simulink model "Bomb"  (R2014a)
settings: Solver=ode45  StartTime=0.0  StopTime=30  RelTol=1e-3
settings Model: Creator=pc32  LastModifiedBy=marwan
settings DebuggingCC: UnderspecifiedInitializationDetection=Classic  StateNameClashWarn=warning

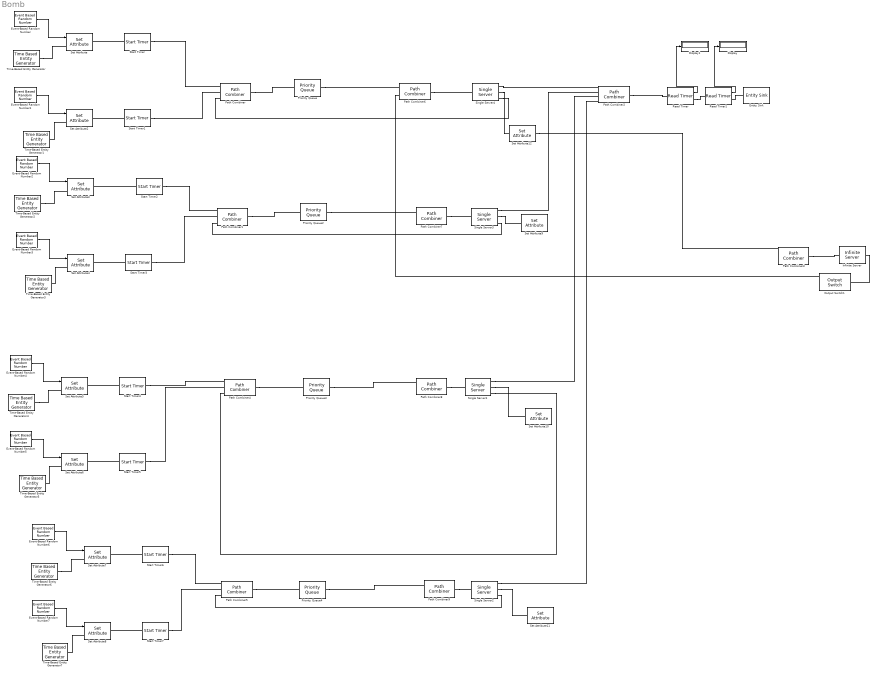
== system Bomb ==
  Display : Display
  Display1 : Display
  Entity Sink : EntitySink
  Event-Based Random Number : EventBasedRandomNumber  meanExp=1/100  Seed=40859
  Event-Based Random Number1 : EventBasedRandomNumber  meanExp=1/100  Seed=94546
  Event-Based Random Number2 : EventBasedRandomNumber  meanExp=1/100  Seed=3
  Event-Based Random Number3 : EventBasedRandomNumber  meanExp=1/100  Seed=4
  Event-Based Random Number4 : EventBasedRandomNumber  meanExp=1/100  Seed=44076
  Event-Based Random Number5 : EventBasedRandomNumber  meanExp=1/100  Seed=5
  Event-Based Random Number6 : EventBasedRandomNumber  meanExp=1/100  Seed=6
  Event-Based Random Number7 : EventBasedRandomNumber  meanExp=1/100  Seed=7
  Infinite Server : InfiniteServer  ServiceTime=0
  Output Switch1 : OutputSwitch  NumberOutputPorts=5  AttributeName=type
  Path Combiner{,1,4..5} (4 alike) : PathCombiner
  Path Combiner2 : PathCombiner  NumberInputPorts=4
  Path Combiner3 : PathCombiner  NumberInputPorts=4
  Path Combiner{6..9} (4 alike) : PathCombiner  NumberInputPorts=2
  Priority Queue{,2..4} (4 alike) : PriorityQueue  Capacity=inf  SortingAttributeName=priority
  Read Timer : ReadTimer  TimerTag=TP  TimerModeOption=Ignore  StatAverageTimeElapsed=on
      settings: OutputPortMap=o3
  Read Timer1 : ReadTimer  TimerTag=TS  TimerModeOption=Ignore  StatAverageTimeElapsed=on
      settings: OutputPortMap=o3
  Set Attribute{,3,5,7} (4 alike) : SetAttribute  AttributeName=ServTime|priority  AttributeFrom=Signal port|Dialog  AttributeValue=1|1  AttributeTreatAsVector=1|1  EvaluatedAttributeValue={ [];1}
  Set Attribute10 : SetAttribute  AttributeName=ch  AttributeValue=3  EvaluatedAttributeValue={ 3}
  Set Attribute11 : SetAttribute  AttributeName=ch  AttributeValue=4  EvaluatedAttributeValue={ 4}
  Set Attribute12 : SetAttribute  AttributeName=ch|priority  AttributeFrom=Dialog|Dialog  AttributeValue=1|2  AttributeTreatAsVector=1|1  EvaluatedAttributeValue={ 1;2}
  Set Attribute{2,4,6,8} (4 alike) : SetAttribute  AttributeName=ServTime|priority  AttributeFrom=Signal port|Dialog  AttributeValue=1|3  AttributeTreatAsVector=1|1  EvaluatedAttributeValue={ [];3}
  Set Attribute9 : SetAttribute  AttributeName=ch  AttributeValue=2  EvaluatedAttributeValue={ 2}
  Single Server{1..4} (4 alike) : SingleServer  ServiceTimeFrom=Attribute  ServiceTime=0  AttributeName=ServTime  PermitPreemption=on  SortingAttributeName=priority  WriteToAttribute=on  ResidualAttributeName=ServTime  EnableTOPort=on
  Start Timer{,2,4,6} (4 alike) : StartTimer  TimerTag=TP  TimerStartedOption=Continue
  Start Timer{1,3,5,7} (4 alike) : StartTimer  TimerTag=TS  TimerStartedOption=Continue
  Time-Based Entity Generator : TimeBasedEntityGenerator  Distribution=Exponential  InitialSeed=11
  Time-Based Entity Generator1 : TimeBasedEntityGenerator  Distribution=Exponential  InitialSeed=12
  Time-Based Entity Generator2 : TimeBasedEntityGenerator  Distribution=Exponential  InitialSeed=13
  Time-Based Entity Generator3 : TimeBasedEntityGenerator  Distribution=Exponential  InitialSeed=14
  Time-Based Entity Generator4 : TimeBasedEntityGenerator  Distribution=Exponential  InitialSeed=15
  Time-Based Entity Generator5 : TimeBasedEntityGenerator  Distribution=Exponential  InitialSeed=16
  Time-Based Entity Generator6 : TimeBasedEntityGenerator  Distribution=Exponential  InitialSeed=17
  Time-Based Entity Generator7 : TimeBasedEntityGenerator  Distribution=Exponential  InitialSeed=18
  wires:
  Event-Based Random Number/1 -> Set Attribute/1
  Event-Based Random Number1/1 -> Set Attribute2/1
  Event-Based Random Number2/1 -> Set Attribute3/1
  Event-Based Random Number3/1 -> Set Attribute4/1
  Event-Based Random Number4/1 -> Set Attribute5/1
  Event-Based Random Number5/1 -> Set Attribute6/1
  Event-Based Random Number6/1 -> Set Attribute7/1
  Event-Based Random Number7/1 -> Set Attribute8/1
  Read Timer/1 -> Display1/1
  Read Timer1/1 -> Display/1
  connections:
  Start Timer/LConn1 -- Set Attribute/RConn1
  Time-Based Entity Generator/RConn1 -- Set Attribute/LConn1
  Time-Based Entity Generator1/RConn1 -- Set Attribute2/LConn1
  Start Timer1/LConn1 -- Set Attribute2/RConn1
  Read Timer/RConn1 -- Read Timer1/LConn1
  Read Timer1/RConn1 -- Entity Sink/LConn1
  Path Combiner2/RConn1 -- Read Timer/LConn1
  Time-Based Entity Generator3/RConn1 -- Set Attribute4/LConn1
  Time-Based Entity Generator2/RConn1 -- Set Attribute3/LConn1
  Start Timer2/LConn1 -- Set Attribute3/RConn1
  Start Timer3/LConn1 -- Set Attribute4/RConn1
  Time-Based Entity Generator5/RConn1 -- Set Attribute6/LConn1
  Time-Based Entity Generator4/RConn1 -- Set Attribute5/LConn1
  Start Timer4/LConn1 -- Set Attribute5/RConn1
  Start Timer5/LConn1 -- Set Attribute6/RConn1
  Time-Based Entity Generator7/RConn1 -- Set Attribute8/LConn1
  Time-Based Entity Generator6/RConn1 -- Set Attribute7/LConn1
  Start Timer6/LConn1 -- Set Attribute7/RConn1
  Start Timer7/LConn1 -- Set Attribute8/RConn1
  Start Timer/RConn1 -- Path Combiner/LConn1
  Start Timer1/RConn1 -- Path Combiner/LConn2
  Path Combiner/RConn1 -- Priority Queue/LConn1
  Start Timer2/RConn1 -- Path Combiner1/LConn1
  Start Timer3/RConn1 -- Path Combiner1/LConn2
  Start Timer4/RConn1 -- Path Combiner4/LConn1
  Start Timer5/RConn1 -- Path Combiner4/LConn2
  Start Timer6/RConn1 -- Path Combiner5/LConn1
  Start Timer7/RConn1 -- Path Combiner5/LConn2
  Path Combiner1/RConn1 -- Priority Queue2/LConn1
  Path Combiner4/RConn1 -- Priority Queue3/LConn1
  Path Combiner5/RConn1 -- Priority Queue4/LConn1
  Single Server4/RConn1 -- Path Combiner2/LConn1
  Single Server3/RConn1 -- Path Combiner2/LConn2
  Single Server1/RConn1 -- Path Combiner2/LConn3
  Single Server2/RConn1 -- Path Combiner2/LConn4
  Single Server4/RConn2 -- Set Attribute12/LConn1
  Single Server3/RConn2 -- Set Attribute9/LConn1
  Single Server1/RConn2 -- Set Attribute10/LConn1
  Single Server2/RConn2 -- Set Attribute11/LConn1
  Path Combiner6/RConn1 -- Single Server4/LConn1
  Priority Queue/RConn1 -- Path Combiner6/LConn1
  Path Combiner7/RConn1 -- Single Server3/LConn1
  Priority Queue2/RConn1 -- Path Combiner7/LConn1
  Path Combiner8/RConn1 -- Single Server1/LConn1
  Priority Queue3/RConn1 -- Path Combiner8/LConn1
  Path Combiner9/RConn1 -- Single Server2/LConn1
  Priority Queue4/RConn1 -- Path Combiner9/LConn1
  Set Attribute12/RConn1 -- Path Combiner3/LConn1
  Output Switch1/RConn1 -- Path Combiner6/LConn2
  Single Server4/RConn3 -- Path Combiner/LConn3
  Path Combiner3/RConn1 -- Infinite Server/LConn1
  Infinite Server/RConn1 -- Output Switch1/LConn1
  Single Server3/RConn3 -- Path Combiner1/LConn3
  Single Server1/RConn3 -- Path Combiner4/LConn3
  Single Server2/RConn3 -- Path Combiner5/LConn3
